simulink model "ThreeTankSIM"  (R2023a)
settings: Solver=ode5  StartTime=0.0  StopTime=300  FixedStep=0.1  MaxStep=0.1  RelTol=1e-5  EnableMultiTasking=on
values from neighbouring files (symbols this model uses):
  C = [1  0  0; 0  1  0]    [LinearModel.mat]
  Hlimit = 350    [Initialise_MiniThreetank_System_A.m]    (also in Initialise_MiniThreetank_System_C.m; Initialise_MiniThreetank_System_D.m; Initialise_MiniThreetank_System_H.m)
  Qlimit = 20    [Initialise_MiniThreetank_System_A.m]    (also in Initialise_MiniThreetank_System_C.m; Initialise_MiniThreetank_System_D.m; Initialise_MiniThreetank_System_H.m)
undefined symbols (not defined in the file or in its folder): a0, ac, b0, bc, G12, G1o, G2o, G32, G3o, Kr, Kx
libraries: simulink x1
settings Model: Creator=ksto036  LastModifiedBy=bl4ck
settings SolverCC: AlgebraicLoopSolver=TrustRegion
settings DataIOCC: SaveFormat=Array  SignalLoggingSaveFormat=ModelDataLogs  SaveOutput=off  SignalLogging=off  SaveTime=off  ReturnWorkspaceOutputs=off
settings OptimizationCC: ReuseModelBlockBuffer=off  ExpressionDepthLimit=2147483647  InitFltsAndDblsToZero=on  LifeSpan=inf
settings DebuggingCC: SaveWithParameterizedLinksMsg=none  UnderspecifiedInitializationDetection=Classic  MergeDetectMultiDrivingBlocksExec=none  SignalResolutionControl=TryResolveAllWithWarning  SolverPrmCheckMsg=warning  MultiTaskDSMMsg=warning  MultiTaskCondExecSysMsg=none  FcnCallInpInsideContextMsg=warning  UnconnectedInputMsg=warning  UnconnectedOutputMsg=warning  UnconnectedLineMsg=warning  AllowSymbolicDim=off  StateNameClashWarn=warning  SFUnexpectedBacktrackingDiag=warning  SFNoUnconditionalDefaultTransitionDiag=warning  SFExecutionAtInitializationDiag=none  ArithmeticOperatorsInVariantConditions=warning
settings HardwareCC: ProdBitPerPointer=32  ProdBitPerSizeT=32  ProdBitPerPtrDiffT=32  ProdLargestAtomicFloat=None  ProdIntDivRoundTo=Undefined  ProdEndianess=Unspecified  ProdWordSize=32  ProdHWDeviceType=32-bit Generic
settings ModelReferenceCC: EnableRefExpFcnMdlSchedulingChecks=on  PropagateSignalLabelsOutOfModel=off
settings SFSimCC: SimUseLocalCustomCode=off  CustomCodeUndefinedFunction=UseInterfaceOnly
settings RTWCC: RTWUseLocalCustomCode=off
settings CodeAppCC: StateflowObjectComments=on
settings GRTTargetCC: TargetFcnLib=ansi_tfl_tmw.mat  TargetLangStandard=C89/C90 (ANSI)  CombineOutputUpdateFcns=off  GRTInterface=on
settings ConfigComp: CovMetricSettings=dw  CovSaveCumulativeToWorkspaceVar=on  CovSaveSingleToWorkspaceVar=on  CovExternalEMLEnable=off

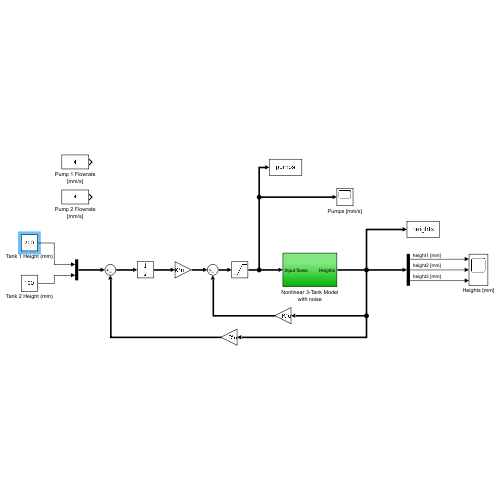
[thumbnail: Simulink's stored preview of the top-level diagram]
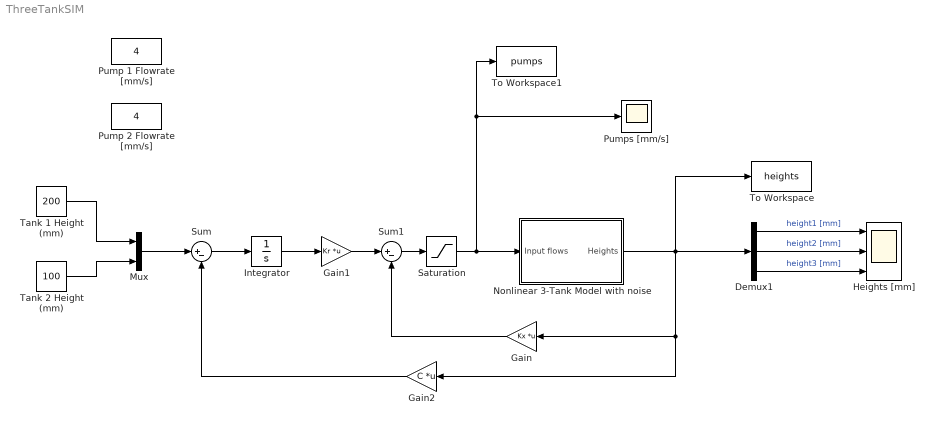
== system ThreeTankSIM ==
  Demux1 : Demux  Outputs=3
  Gain : Gain  Gain=Kx  Multiplication=Matrix(K*u)
  Gain1 : Gain  Gain=Kr  Multiplication=Matrix(K*u)
  Gain2 : Gain  Gain=C  Multiplication=Matrix(K*u)
  Heights [mm] : Scope  NumInputPorts=3
  Integrator : Integrator
  Mux : Mux  Inputs=2
  Nonlinear 3-Tank Model with noise : Subsystem
  Pump 1 Flowrate [mm/s] : Constant  Value=4
  Pump 2 Flowrate [mm/s] : Constant  Value=4
  Pumps [mm/s] : Scope
  Saturation : Saturate  UpperLimit=Qlimit  LowerLimit=0  LinearizeAsGain=off
  Sum : Sum  Inputs=|+-
  Sum1 : Sum  Inputs=|+-
  Tank 1 Height (mm) : Constant  Value=200
  Tank 2 Height (mm) : Constant  Value=100
  To Workspace : ToWorkspace  VariableName=heights  SaveFormat=Structure With Time  SampleTime=-1
  To Workspace1 : ToWorkspace  VariableName=pumps  SaveFormat=Structure With Time  SampleTime=-1
  wires:
  Demux1/3 -> Heights [mm]/3  "height3 [mm]"
  Demux1/2 -> Heights [mm]/2  "height2 [mm]"
  Demux1/1 -> Heights [mm]/1  "height1 [mm]"
  Nonlinear 3-Tank Model with noise/1(Heights) -> Gain2/1, Gain/1, To Workspace/1, Demux1/1
  Saturation/1 -> Nonlinear 3-Tank Model with noise/1(Input flows), Pumps [mm/s]/1, To Workspace1/1
  Tank 1 Height (mm)/1 -> Mux/1
  Tank 2 Height (mm)/1 -> Mux/2
  Mux/1 -> Sum/1
  Gain1/1 -> Sum1/1
  Integrator/1 -> Gain1/1
  Sum/1 -> Integrator/1
  Gain/1 -> Sum1/2
  Sum1/1 -> Saturation/1
  Gain2/1 -> Sum/2

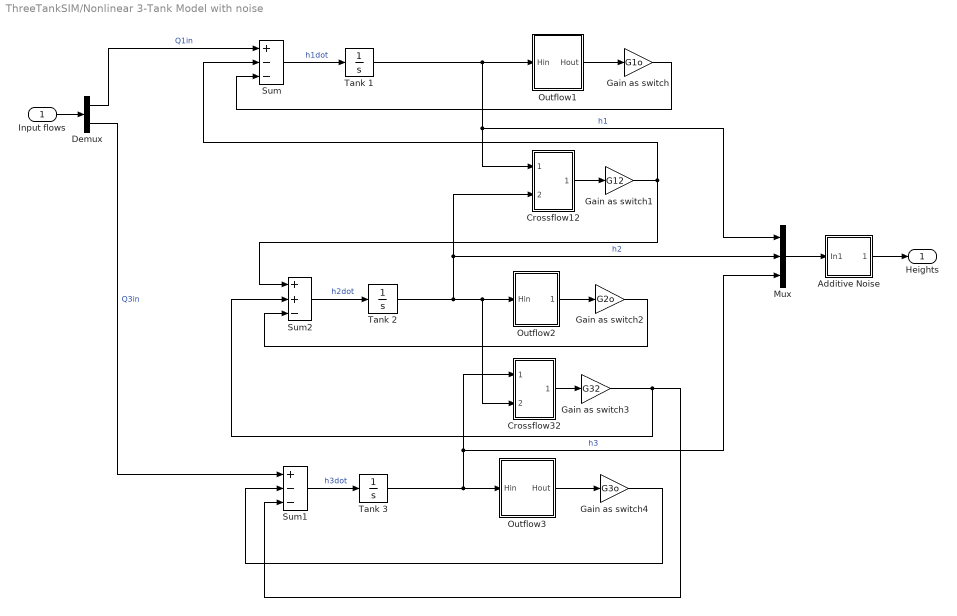
== system ThreeTankSIM/Nonlinear 3-Tank Model with noise ==
  Input flows : Inport
  Additive Noise : Subsystem
  Crossflow12 : Subsystem
  Crossflow32 : Subsystem
  Demux : Demux  Outputs=2
      settings: DisplayOption=none
  Gain as switch : Gain  Gain=G1o  SaturateOnIntegerOverflow=on  OutDataTypeStr=Inherit: Same as input  ParamDataTypeStr=Inherit: Same as input
  Gain as switch1 : Gain  Gain=G12  SaturateOnIntegerOverflow=on  OutDataTypeStr=Inherit: Same as input  ParamDataTypeStr=Inherit: Same as input
  Gain as switch2 : Gain  Gain=G2o  SaturateOnIntegerOverflow=on  OutDataTypeStr=Inherit: Same as input  ParamDataTypeStr=Inherit: Same as input
  Gain as switch3 : Gain  Gain=G32  SaturateOnIntegerOverflow=on  OutDataTypeStr=Inherit: Same as input  ParamDataTypeStr=Inherit: Same as input
  Gain as switch4 : Gain  Gain=G3o  SaturateOnIntegerOverflow=on  OutDataTypeStr=Inherit: Same as input  ParamDataTypeStr=Inherit: Same as input
  Mux : Mux  Inputs=3
  Outflow1 : Subsystem
  Outflow2 : Subsystem
  Outflow3 : Subsystem
  Sum : Sum  Inputs=+--  SaturateOnIntegerOverflow=on
  Sum1 : Sum  Inputs=+--  SaturateOnIntegerOverflow=on
  Sum2 : Sum  Inputs=++-  SaturateOnIntegerOverflow=on
  Tank 1 : Integrator  LimitOutput=on  UpperSaturationLimit=Hlimit  LowerSaturationLimit=0
  Tank 2 : Integrator  LimitOutput=on  UpperSaturationLimit=Hlimit  LowerSaturationLimit=0
  Tank 3 : Integrator  LimitOutput=on  UpperSaturationLimit=Hlimit  LowerSaturationLimit=0
  Heights : Outport  VectorParamsAs1DForOutWhenUnconnected=off
  wires:
  Mux/1 -> Additive Noise/1(In1)
  Demux/1 -> Sum/1  "Q1in"
  Input flows/1 -> Demux/1
  Gain as switch/1 -> Sum/3
  Outflow1/1(Hout) -> Gain as switch/1
  Gain as switch1/1 -> Sum/2, Sum2/1
  Crossflow12/1(Out1) -> Gain as switch1/1
  Gain as switch2/1 -> Sum2/3
  Outflow2/1(Hout) -> Gain as switch2/1
  Gain as switch3/1 -> Sum2/2, Sum1/3
  Crossflow32/1(Out1) -> Gain as switch3/1
  Gain as switch4/1 -> Sum1/2
  Outflow3/1(Hout) -> Gain as switch4/1
  Tank 3/1 -> Mux/3, Crossflow32/1(In1), Outflow3/1(Hin)  "h3"
  Tank 2/1 -> Mux/2, Crossflow12/2(In2), Crossflow32/2(In2), Outflow2/1(Hin)  "h2"
  Tank 1/1 -> Mux/1, Crossflow12/1(In1), Outflow1/1(Hin)  "h1"
  Demux/2 -> Sum1/1  "Q3in"
  Sum2/1 -> Tank 2/1  "h2dot"
  Sum1/1 -> Tank 3/1  "h3dot"
  Sum/1 -> Tank 1/1  "h1dot"
  Additive Noise/1(Out1) -> Heights/1

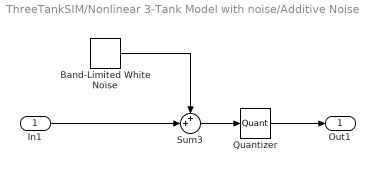
== system ThreeTankSIM/Nonlinear 3-Tank Model with noise/Additive Noise ==
  In1 : Inport
  Band-Limited White Noise : simulink/Sources/Band-Limited White Noise  Cov=[0.002]  Ts=0.1  seed=[23341]
  Quantizer : Quantizer  QuantizationInterval=0.2
  Sum3 : Sum  Inputs=++|  SaturateOnIntegerOverflow=on
  Out1 : Outport  VectorParamsAs1DForOutWhenUnconnected=off
  wires:
  Quantizer/1 -> Out1/1
  Band-Limited White Noise/1 -> Sum3/1
  Sum3/1 -> Quantizer/1
  In1/1 -> Sum3/2

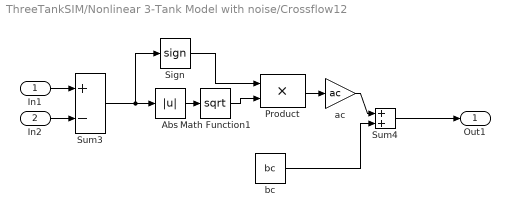
== system ThreeTankSIM/Nonlinear 3-Tank Model with noise/Crossflow12 ==
  In1 : Inport
  In2 : Inport  Port=2
  Abs : Abs
  Math Function1 : Math  Operator=sqrt  SignedPower=on
  Product : Product  SaturateOnIntegerOverflow=on  OutDataTypeStr=Inherit: Same as first input
  Sign : Signum
  Sum3 : Sum  Inputs=+-  SaturateOnIntegerOverflow=on
  Sum4 : Sum  SaturateOnIntegerOverflow=on
  ac : Gain  Gain=ac  SaturateOnIntegerOverflow=on  OutDataTypeStr=Inherit: Same as input  ParamDataTypeStr=Inherit: Same as input
  bc : Constant  Value=bc
  Out1 : Outport  VectorParamsAs1DForOutWhenUnconnected=off
  wires:
  Sum4/1 -> Out1/1
  In2/1 -> Sum3/2
  In1/1 -> Sum3/1
  Product/1 -> ac/1
  Math Function1/1 -> Product/2
  Sign/1 -> Product/1
  Abs/1 -> Math Function1/1
  ac/1 -> Sum4/1
  bc/1 -> Sum4/2
  Sum3/1 -> Sign/1, Abs/1

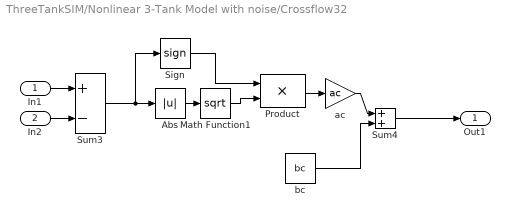
== system ThreeTankSIM/Nonlinear 3-Tank Model with noise/Crossflow32 ==
  In1 : Inport
  In2 : Inport  Port=2
  Abs : Abs
  Math Function1 : Math  Operator=sqrt  SignedPower=on
  Product : Product  SaturateOnIntegerOverflow=on  OutDataTypeStr=Inherit: Same as first input
  Sign : Signum
  Sum3 : Sum  Inputs=+-  SaturateOnIntegerOverflow=on
  Sum4 : Sum  SaturateOnIntegerOverflow=on
  ac : Gain  Gain=ac  SaturateOnIntegerOverflow=on  OutDataTypeStr=Inherit: Same as input  ParamDataTypeStr=Inherit: Same as input
  bc : Constant  Value=bc
  Out1 : Outport  VectorParamsAs1DForOutWhenUnconnected=off
  wires:
  Sum4/1 -> Out1/1
  In2/1 -> Sum3/2
  In1/1 -> Sum3/1
  Product/1 -> ac/1
  Math Function1/1 -> Product/2
  Sign/1 -> Product/1
  Abs/1 -> Math Function1/1
  ac/1 -> Sum4/1
  bc/1 -> Sum4/2
  Sum3/1 -> Sign/1, Abs/1

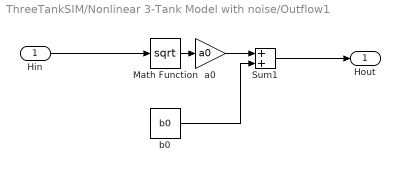
== system ThreeTankSIM/Nonlinear 3-Tank Model with noise/Outflow1 ==
  Hin : Inport
  Math Function : Math  Operator=sqrt  SignedPower=on
  Sum1 : Sum  SaturateOnIntegerOverflow=on
  a0 : Gain  Gain=a0  SaturateOnIntegerOverflow=on  OutDataTypeStr=Inherit: Same as input  ParamDataTypeStr=Inherit: Same as input
  b0 : Constant  Value=b0
  Hout : Outport  VectorParamsAs1DForOutWhenUnconnected=off
  wires:
  Sum1/1 -> Hout/1
  Hin/1 -> Math Function/1
  a0/1 -> Sum1/1
  b0/1 -> Sum1/2
  Math Function/1 -> a0/1

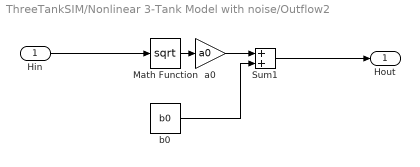
== system ThreeTankSIM/Nonlinear 3-Tank Model with noise/Outflow2 ==
  Hin : Inport
  Math Function : Math  Operator=sqrt  SignedPower=on
  Sum1 : Sum  SaturateOnIntegerOverflow=on
  a0 : Gain  Gain=a0  SaturateOnIntegerOverflow=on  OutDataTypeStr=Inherit: Same as input  ParamDataTypeStr=Inherit: Same as input
  b0 : Constant  Value=b0
  Hout : Outport  VectorParamsAs1DForOutWhenUnconnected=off
  wires:
  Sum1/1 -> Hout/1
  Hin/1 -> Math Function/1
  a0/1 -> Sum1/1
  b0/1 -> Sum1/2
  Math Function/1 -> a0/1

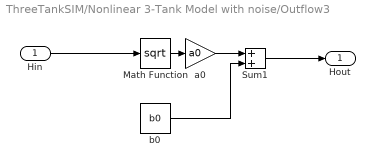
== system ThreeTankSIM/Nonlinear 3-Tank Model with noise/Outflow3 ==
  Hin : Inport
  Math Function : Math  Operator=sqrt  SignedPower=on
  Sum1 : Sum  SaturateOnIntegerOverflow=on
  a0 : Gain  Gain=a0  SaturateOnIntegerOverflow=on  OutDataTypeStr=Inherit: Same as input  ParamDataTypeStr=Inherit: Same as input
  b0 : Constant  Value=b0
  Hout : Outport  VectorParamsAs1DForOutWhenUnconnected=off
  wires:
  Sum1/1 -> Hout/1
  Hin/1 -> Math Function/1
  a0/1 -> Sum1/1
  b0/1 -> Sum1/2
  Math Function/1 -> a0/1
